simulink model "FlexSensor_4in5_v1"  (R2017b)
settings: Solver=VariableStepAuto  StartTime=0.0  StopTime=inf  RelTol=1e-3
libraries: fl_lib x8, nesl_utility x7
settings Model: Creator=stark  LastModifiedBy=stark

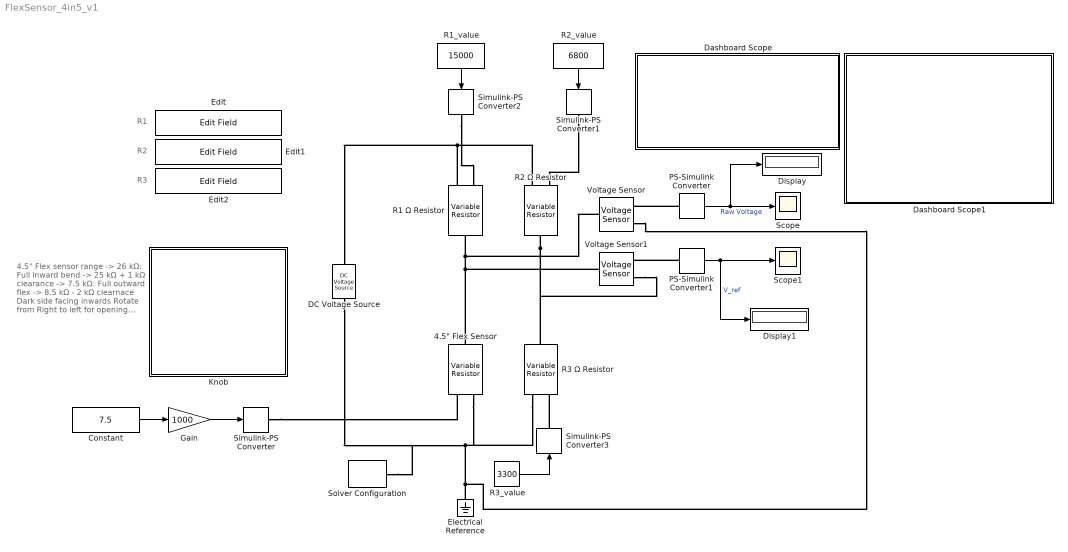
== system FlexSensor_4in5_v1 ==
  note: R2
  note: R3
  note: 4.5" Flex sensor range
      | -> 26 kΩ: Full inward bend
      | -> 25 kΩ + 1 kΩ clearance
      | -> 7.5 kΩ: Full outward flex
      | -> 8.5 kΩ - 2 kΩ clearnace
      | Dark side facing inwards
      | Rotate from Right to left for
      | opening outwards and Left
      | to right for clentching inwards
  note: R1
  "4.5\" Flex Sensor" : fl_lib/Electrical/Electrical Elements/Variable Resistor  Rmin=0 Ohm  i_specify=off  i_priority=None  i=0 A  i_nominal_specify=off  i_nominal_unit=A  i_nominal_value=1  v_specify=off  v_priority=None  v=0 V  v_nominal_specify=off  v_nominal_unit=V  v_nominal_value=1
  Constant : Constant  Value=7.5
  DC Voltage Source : fl_lib/Electrical/Electrical Sources/DC Voltage Source  v0=5 V
  Dashboard Scope : Subsystem  DialogController=hmiCreateDDGDialog  IsWebBlock=on  mask(MWDashboardBlock){webBlockId=1b419ccd-0990-40aa-b9e6-846dc053495d, webBlockType=sdiscope, ShowInitialText=on, HMISrcModelName=FlexSensor_4in5_v1}
      mask prompts: webBlockId "WebBlock Id"; webBlockType "WebBlock Type"; HMISrcModelName "Source Model"
      mask help: SimulinkHMI:dialogs:HMIScopeDialogDesc
      mask Help: helpview([docroot '/mapfiles/simulink.map'], 'hmi_scope')
      mask Display:
      | if strcmp(get_param(bdroot(gcb),'BlockDiagramType'), 'library')
      |     image([(matlabroot) '/toolbox/simulink/hmi/icons/DashboardScope.png']);
      | end
  Dashboard Scope1 : Subsystem  DialogController=hmiCreateDDGDialog  IsWebBlock=on  mask(MWDashboardBlock){webBlockId=24330aa9-d2bc-4372-9a70-c3e86f4a543e, webBlockType=sdiscope, ShowInitialText=on, HMISrcModelName=FlexSensor_4in5_v1}
      mask prompts: webBlockId "WebBlock Id"; webBlockType "WebBlock Type"; HMISrcModelName "Source Model"
      mask help: SimulinkHMI:dialogs:HMIScopeDialogDesc
      mask Help: helpview([docroot '/mapfiles/simulink.map'], 'hmi_scope')
      mask Display:
      | if strcmp(get_param(bdroot(gcb),'BlockDiagramType'), 'library')
      |     image([(matlabroot) '/toolbox/simulink/hmi/icons/DashboardScope.png']);
      | end
  Display : Display
  Display1 : Display
  Edit : EditField  WebBlockId=8  ModelName=FlexSensor_2in2_v1  LabelPosition=Hide  ShowInitialText=off  Alignment=Center
  Edit1 : EditField  WebBlockId=9  ModelName=FlexSensor_2in2_v1  LabelPosition=Hide  ShowInitialText=off  Alignment=Center
  Edit2 : EditField  WebBlockId=10  ModelName=FlexSensor_2in2_v1  LabelPosition=Hide  ShowInitialText=off  Alignment=Center
  Electrical Reference : fl_lib/Electrical/Electrical Elements/Electrical Reference
  Gain : Gain  Gain=1000
  Knob : Subsystem  DialogController=hmiCreateDDGDialog  IsWebBlock=on  mask(MWDashboardBlock){webBlockId=85848859-5c60-4759-b489-606f39201498, webBlockType=continuousknob, ShowInLibBrowser=on, ShowInitialText=on, HMISrcModelName=FlexSensor_4in5_v1}
      mask prompts: webBlockId "WebBlock Id"; webBlockType "WebBlock Type"; HMISrcModelName "Source Model"
      mask help: SimulinkHMI:dialogs:ContinuousKnobDialogDesc
      mask Help: helpview([docroot '/mapfiles/simulink.map'], 'hmi_knob')
      mask Display:
      | if strcmp(get_param(bdroot(gcb),'BlockDiagramType'), 'library')
      |     image([(matlabroot) '/toolbox/simulink/hmi/icons/ContinuousKnob.png']);
      | end
  PS-Simulink Converter : nesl_utility/PS-Simulink Converter  PhysicalDomain=network_engine_domain  SubClassName=ps_output  LeftPortType=input  RightPortType=output  PseudoPeriodic=off  Frequencies=[]  Unit=1  AffineConversion=off
  PS-Simulink Converter1 : nesl_utility/PS-Simulink Converter  PhysicalDomain=network_engine_domain  SubClassName=ps_output  LeftPortType=input  RightPortType=output  PseudoPeriodic=off  Frequencies=[]  Unit=1  AffineConversion=off
  R1 Ω Resistor : fl_lib/Electrical/Electrical Elements/Variable Resistor  Rmin=0 Ohm  i_specify=off  i_priority=None  i=0 A  i_nominal_specify=off  i_nominal_unit=A  i_nominal_value=1  v_specify=off  v_priority=None  v=0 V  v_nominal_specify=off  v_nominal_unit=V  v_nominal_value=1
  R1_value : Constant  Value=15000
  R2 Ω Resistor : fl_lib/Electrical/Electrical Elements/Variable Resistor  Rmin=0 Ohm  i_specify=off  i_priority=None  i=0 A  i_nominal_specify=off  i_nominal_unit=A  i_nominal_value=1  v_specify=off  v_priority=None  v=0 V  v_nominal_specify=off  v_nominal_unit=V  v_nominal_value=1
  R2_value : Constant  Value=6800
  R3 Ω Resistor : fl_lib/Electrical/Electrical Elements/Variable Resistor  Rmin=0 Ohm  i_specify=off  i_priority=None  i=0 A  i_nominal_specify=off  i_nominal_unit=A  i_nominal_value=1  v_specify=off  v_priority=None  v=0 V  v_nominal_specify=off  v_nominal_unit=V  v_nominal_value=1
  R3_value : Constant  Value=3300
  Scope : Scope
  Scope1 : Scope
  Simulink-PS Converter{,1..3} (4 alike) : nesl_utility/Simulink-PS Converter  PhysicalDomain=network_engine_domain  SubClassName=ps_input  LeftPortType=input  RightPortType=output  PseudoPeriodic=off  Frequencies=[]  NoiseDistribution=none  NoiseParameters=[]  Unit=1  AffineConversion=off  FilteringAndDerivatives=provide  SimscapeFilterOrder=1  InputFilterTimeConstant=0.001  UdotUserProvided=0
  Solver Configuration : nesl_utility/Solver Configuration  PhysicalDomain=network_engine_domain  SubClassName=solver  LeftPortType=input  RightPortType=generic  Accelerate=off  Tones=[]  Harmonics=[]  SimulateNoise=off  Profile=off  UseLocalSampling=off  EnableSwitchedLinearOptims=on  FrequencyDomain=off  UseCCode=off  RelTol=0.001  AbsTol=1e-06  MinStep=1e-09  ToWorkspace=off  RevertToSquareIcSolve=off  NumHomotopyIterations=100  PhasorMode=off  PhasorModeNumHarmonics=1  DoDC=off  ResidualTolerance=1e-09  UseLocalSolver=off  LocalSolverChoice=NE_BACKWARD_EULER_ADVANCER  LocalSolverSampleTime=0.001  DoFixedCost=off  MaxNonlinIter=3  MaxModeIter=2  LinearAlgebra=Sparse  DelaysMemoryBudget=1024  AutomaticFiltering=on  FilteringTimeConstant=0.001
  Voltage Sensor : fl_lib/Electrical/Electrical Sensors/Voltage Sensor
  Voltage Sensor1 : fl_lib/Electrical/Electrical Sensors/Voltage Sensor
  wires:
  R2_value/1 -> Simulink-PS Converter1/1
  R1_value/1 -> Simulink-PS Converter2/1
  PS-Simulink Converter1/1 -> Display1/1, Scope1/1  "V_ref"
  R3_value/1 -> Simulink-PS Converter3/1
  Gain/1 -> Simulink-PS Converter/1
  Constant/1 -> Gain/1
  PS-Simulink Converter/1 -> Display/1, Scope/1  "Raw Voltage"
  connections:
  R2 Ω Resistor/LConn2 -- R1 Ω Resistor/LConn2 -- DC Voltage Source/LConn1
  Electrical Reference/LConn1 -- "4.5\" Flex Sensor"/LConn2 -- R3 Ω Resistor/LConn2 -- DC Voltage Source/RConn1 -- Solver Configuration/RConn1 -- Voltage Sensor/RConn2
  R2 Ω Resistor/RConn1 -- R3 Ω Resistor/RConn1 -- Voltage Sensor1/RConn2
  PS-Simulink Converter1/LConn1 -- Voltage Sensor1/RConn1
  Simulink-PS Converter3/RConn1 -- R3 Ω Resistor/LConn1
  PS-Simulink Converter/LConn1 -- Voltage Sensor/RConn1
  Simulink-PS Converter2/RConn1 -- R1 Ω Resistor/LConn1
  Simulink-PS Converter/RConn1 -- "4.5\" Flex Sensor"/LConn1
  Simulink-PS Converter1/RConn1 -- R2 Ω Resistor/LConn1
  "4.5\" Flex Sensor"/RConn1 -- Voltage Sensor1/LConn1 -- R1 Ω Resistor/RConn1 -- Voltage Sensor/LConn1

== system FlexSensor_4in5_v1/Dashboard Scope ==

== system FlexSensor_4in5_v1/Dashboard Scope1 ==

== system FlexSensor_4in5_v1/Knob ==
